simulink model "S_EXP_PI_MPPT_V1"  (R2017a)
settings: Solver=FixedStepDiscrete  StartTime=0.0  StopTime=10.0  RelTol=1e-3  EnableMultiTasking=on
undefined symbols (not defined in the file or in its folder): Down, GPTRIP1SEL, GPTRIP2SEL, TZ1, TZ2, Up
libraries: c2802xlib x3, c2806xlib x2, c280xlib x2, simulink x1, c2000lib x1
settings Model: ExtModeTrigDuration=8  Creator=dricl  LastModifiedBy=dricl
settings OptimizationCC: DefaultUnderspecifiedDataType=single  PassReuseOutputArgsAs=Individual arguments  MaxStackSize=512
settings DebuggingCC: ParameterTunabilityLossMsg=error
settings HardwareCC: ProdBitPerChar=16  ProdBitPerInt=16  ProdBitPerPointer=32  ProdBitPerSizeT=32  ProdBitPerPtrDiffT=32  ProdLargestAtomicInteger=Integer  ProdLargestAtomicFloat=None  ProdWordSize=16  ProdLongLongMode=on  ProdHWDeviceType=Texas Instruments->C2000
settings SFSimCC: MATLABDynamicMemAlloc=off
settings RTWCC: SystemTargetFile=ert.tlc  HardwareBoard=TI Piccolo F2806x  TLCOptions=-aInlineSetEventsForThisBaseRateFcn=TLC_FALSE -aSuppressMultiTaskScheduler=TLC_FALSE -aRateBasedStepFcn=1  TemplateMakefile=ert_default_tmf  Description=Embedded Coder  Toolchain=Texas Instruments Code Composer Studio v5 (C2000)  CodeExecutionProfiling=on  CodeProfilingSaveOptions=AllData  CodeProfilingInstrumentation=on
settings CodeAppCC: ForceParamTrailComments=on  IgnoreCustomStorageClasses=off  OperatorAnnotations=on  SimulinkDataObjDesc=on  SFDataObjDesc=on  MATLABFcnDesc=on  InsertBlockDesc=on  MATLABSourceComments=on
settings ERTTargetCC: CodeReplacementLibrary=TI C28x  MemSecPackage=tic2000demospkg  MemSecFuncExecute=code_ramfuncs

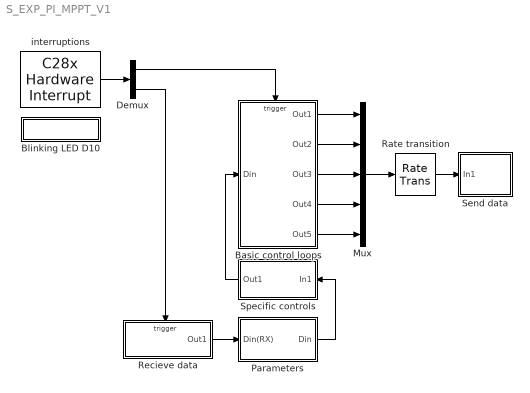
== system S_EXP_PI_MPPT_V1 ==
  Basic control loops : Subsystem  TreatAsAtomicUnit=on
      settings: RTWSystemCode=Nonreusable function
  Blinking LED D10 : Subsystem
  Demux : Demux  Outputs=2
  Mux : Mux  Inputs=5
  Parameters : Subsystem  TreatAsAtomicUnit=on
  Rate transition : RateTransition  Integrity=off  Deterministic=off  OutPortSampleTime=1/5e3
  Recieve data : Subsystem  SystemSampleTime=1e-3
      settings: RTWSystemCode=Nonreusable function
  Send data : Subsystem  TreatAsAtomicUnit=on
  Specific controls : Subsystem  TreatAsAtomicUnit=on
  interruptions : c2000lib/Scheduling/C28x Hardware Interrupt  irqnumbers=[1 9]  pienumbers=[1 1]  irqpriorities=[30 50]  irqpreempts=[1 0]  showinput=off  dspchiptype=C280X
      settings: SourceProductName=Embedded Coder Support Package for Texas Instruments C2000 Processors  SourceProductBaseCode=TIC2000
  wires:
  interruptions/1 -> Demux/1
  Demux/2 -> Recieve data/Trigger
  Recieve data/1(Out1) -> Parameters/1(Din(RX))
  Demux/1 -> Basic control loops/Trigger
  Parameters/1(Din) -> Specific controls/1(In1)
  Specific controls/1(Out1) -> Basic control loops/1(Din)
  Rate transition/1 -> Send data/1(In1)
  Mux/1 -> Rate transition/1
  Basic control loops/1(Out1) -> Mux/1
  Basic control loops/2(Out2) -> Mux/2
  Basic control loops/3(Out3) -> Mux/3
  Basic control loops/4(Out4) -> Mux/4
  Basic control loops/5(Out5) -> Mux/5

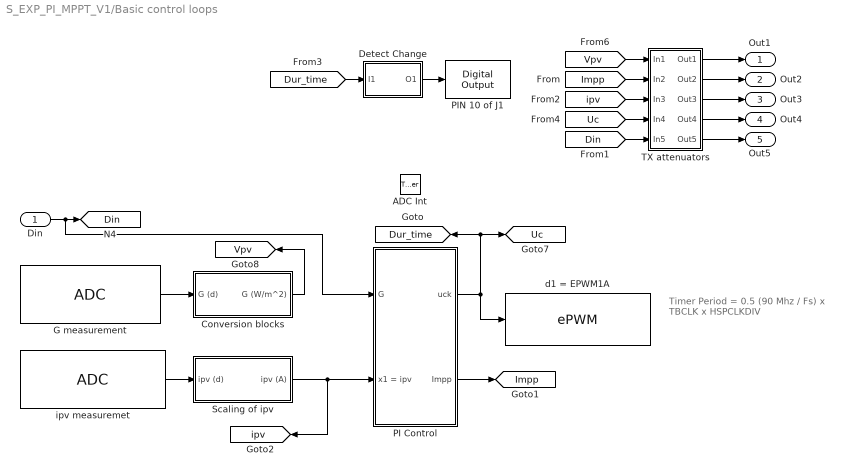
== system S_EXP_PI_MPPT_V1/Basic control loops ==
  note: Timer Period =
      |  0.5 (90 Mhz / Fs)  x
      | TBCLK x HSPCLKDIV
  Din : Inport
  ADC Int : TriggerPort  TriggerType=function-call  VariantControl=Variant
  Conversion blocks : Subsystem  Priority=5  TreatAsAtomicUnit=on
  Detect Change : Subsystem  TreatAsAtomicUnit=on
  G measurement : c2802xlib/ADC  ADCModule=1  samplingMode=Single sample mode  ADCResolution=12-bit (Single-ended input)  useSOC1=SOC1  useSOC2=SOC0_SOC1  SOCAcquisitionWindow=7  SOCTriggerSource=ePWM1_ADCSOCA  SOCInterruptTrigger=No ADCINT  Ts=-1  dType=uint16  postInterrupt=off  interruptSel=ADCINT1  ADCINTContinuous=on  endma=off  chdma=1  blkParamProc=C2000  conv1=ADCINA1  conv2=ADCINA0 and ADCINB0  conv1_Type4=ADCIN0  conv2_Type4=ADCIN0 and ADCIN1
      settings: SourceProductName=Embedded Coder Support Package for Texas Instruments C2000 Processors
  PI Control : Subsystem  Priority=7
  PIN 10 of J1 : c2806xlib/Digital Output  GPIO_Number=GPIO32~GPIO39  GPIO_Bit0=on  GPIO_BIT0_Toggle=off  GPIO_Bit1=off  GPIO_BIT1_Toggle=off  GPIO_Bit2=off  GPIO_BIT2_Toggle=off  GPIO_Bit3=off  GPIO_BIT3_Toggle=off  GPIO_Bit4=off  GPIO_BIT4_Toggle=off  GPIO_Bit5=off  GPIO_BIT5_Toggle=off  GPIO_Bit6=off  GPIO_BIT6_Toggle=off  GPIO_Bit7=off  GPIO_BIT7_Toggle=off
      settings: SourceProductName=Embedded Coder Support Package for Texas Instruments C2000 Processors  SourceProductBaseCode=TIC2000
  Scaling of ipv : Subsystem  Priority=6  TreatAsAtomicUnit=on
  TX attenuators : Subsystem  TreatAsAtomicUnit=on
  d1 = EPWM1A : c2802xlib/ePWM  useModule=ePWM1  ePWMxLINKTBPRD=Not Linked  periodUnits=Clock cycles  timerSource=Specify via dialog  timerPeriod_clk=9000  timerPeriod_sec=0.0001  tbshadow=Counter equals to zero  countingMode=Up-Down  phaseActiveEnable=Disable  phaseDirection=Count down after sync  phaseActive=0  synchronizationEnable=off  dcaevt1Sync=off  dcbevt1Sync=off  synchronizationOption=Disable  clockPrescale=1  HSclockPrescale=1  enswap=off  ePWMxAStatus=on  ePWMxAactionLogic1=Do nothing  ePWMxAactionLogic2=Do nothing  ePWMxAactionLogic3=Clear  ePWMxAactionLogic4=Set  ePWMxAactionLogic5=Do nothing  ePWMxAactionLogic6=Do nothing  ePWMxALoadMode=Load on counter equals to zero (CTR=Zero)  ePWMxACSFenable=off  ePWMxACSFvalue=Forcing disable  ePWMxASFreload=Zero  ePWMxBStatus=off  ePWMxBactionLogic1=Set  ePWMxBactionLogic2=Clear  ePWMxBactionLogic3=Do nothing  ePWMxBactionLogic4=Do nothing  ePWMxBactionLogic5=Clear  ePWMxBactionLogic6=Set  ePWMxBLoadMode=Load on counter equals to zero (CTR=Zero)  ePWMxBCSFenable=off  ePWMxBCSFvalue=Forcing disable  ePWMxBSFreload=Zero  ePWNxBOutWay=off  ePWMxLINKCMPA=Not Linked  CMPAUnits=Clock cycles  CMPASource=Input port  CMPAValue_per=50  CMPAValue_clk=9000/2  enCMPAshadow=Counter equals to zero  ePWMxLINKCMPB=Not Linked  CMPBUnits=Clock cycles  CMPBSource=Specify via dialog  CMPBValue_per=50  CMPBValue_clk=9000/2  enCMPBshadow=Counter equals to zero  ePWMxLINKCMPC=Not Linked  CMPCUnits=Clock cycles  CMPCSource=Specify via dialog  CMPCValue_per=50  CMPCValue_clk=32000  enCMPCshadow=Counter equals to zero  ePWMxLINKCMPD=Not Linked  CMPDUnits=Clock cycles  CMPDSource=Specify via dialog  CMPDValue_per=50  CMPDValue_clk=32000  enCMPDshadow=Counter equals to zero  enableDBePWMxA=on  enableDBePWMxB=on  enhalfcycle=off  DBpolarity=Active high complementary (AHC)  DBedgeDelay=Positive  DBSource_ePWMxA=ePWMxA  DBSource_ePWMxB=ePWMxA  DBperiodSource=Specify via dialog  REDperiod=50  FEDperiod=50  adcstartModuleA=on  adcrequestEventA=First event  adcstartEventA=Counter equals to period (CTR=PRD)  adcstartEventA_type2=Digital Compare Module A Event 1 start of conversion (DCAEVT1.soc)  adcstartModuleB=off  adcrequestEventB=First event  adcstartEventB=Counter equals to zero (CTR=Zero)  adcstartEventB_type2=Counter equals to zero (CTR=Zero)  intEn=off  intPrd=First event  intSel=Counter equals to zero (CTR=Zero)  intSel_type2=Counter equals to zero (CTR=Zero)  hrpe=off  enHRPWM=off  HRPWM_LoadMode=Counter equals to period (CTR=PRD)  HRPWM_CTLMode=Duty or Period control mode  HRPWM_EDGMode=Both edge  hrpeb=off  enHRPWMB=off  HRPWM_LoadModeB=Counter equals to zero (CTR=ZERO)  HRPWM_CTLModeB=Duty or Period control mode  HRPWM_EDGModeB=Both edge  enSFO=on  enautoconv=on  chopperEnable=off  chopperFrequency=1  chopperFirstwidth=1  chopperDuty=12.5%  tripZonesource=Specify via dialog  tzselOSHT1=off  tzselOSHT2=off  tzselOSHT3=off  tzselOSHDCAEV1=off  tzselOSHDCBEV1=off  tzselCBC1=off  tzselCBC2=off  tzselCBC3=off  tzselCBCDCAEV2=off  tzselCBCDCBEV2=off  tzselOSHT4=off  tzselOSHT5=off  tzselOSHT6=off  tzselCBC4=off  tzselCBC5=off  tzselCBC6=off  enTzOstIntr=off  enTzCbcIntr=off  enTzDCAEVT1Intr=off  enTzDCAEVT2Intr=off  enTzDCBEVT1Intr=off  enTzDCBEVT2Intr=off  ePWMxAforced=No action  ePWMxBforced=No action  DCAEVT1forced=No action  DCBEVT1forced=No action  DCAEVT2forced=No action  DCBEVT2forced=No action  dcah=Trip Zone 1 input (TZ1)  dcal=Trip Zone 2 input (TZ2)  dcbh=Trip Zone 1 input (TZ1)  dcbl=Trip Zone 2 input (TZ2)  dcah_type2=GPTRIP1SEL/(TZ1)  dcal_type2=GPTRIP2SEL/(TZ2)  dcbh_type2=GPTRIP1SEL/(TZ1)  dcbl_type2=GPTRIP2SEL/(TZ2)  gendcaevt1=Event disabled  gendcaevt2=Event disabled  gendcbevt1=Event disabled  gendcbevt2=Event disabled  dcaevt1src=DCAEVT1 with sync  dcaevt2src=DCAEVT2 with sync  dcbevt1src=DCBEVT1 with sync  dcbevt2src=DCBEVT2 with sync  pulsesel=Counter equals to zero (CTR=Zero)  blankinv=off  blankoffset=0  blankwidth=0  evsrcsel=Filtered version of DCAEVT1 (DCAEVT1FILT)  encape=off  PwmType=C2000
      settings: SourceProductName=Embedded Coder Support Package for Texas Instruments C2000 Processors
  ipv measuremet : c2802xlib/ADC  ADCModule=1  samplingMode=Single sample mode  ADCResolution=12-bit (Single-ended input)  useSOC1=SOC2  useSOC2=SOC0_SOC1  SOCAcquisitionWindow=7  SOCTriggerSource=ePWM1_ADCSOCA  SOCInterruptTrigger=No ADCINT  Ts=-1  dType=uint16  postInterrupt=on  interruptSel=ADCINT1  ADCINTContinuous=on  endma=off  chdma=1  blkParamProc=C2000  conv1=ADCINA0  conv2=ADCINA0 and ADCINB0  conv1_Type4=ADCIN0  conv2_Type4=ADCIN0 and ADCIN1
      settings: SourceProductName=Embedded Coder Support Package for Texas Instruments C2000 Processors
  Out1 : Outport
  Out2 : Outport  Port=2
  Out3 : Outport  Port=3
  Out4 : Outport  Port=4
  Out5 : Outport  Port=5
  tag scope: Din=global, Dur_time=global, Impp=global, Uc=global, Vpv=global, ipv=global
  wires:
  Din/1 -> PI Control/1(G), [Din]
  ipv measuremet/1 -> Scaling of ipv/1(ipv (d))
  Scaling of ipv/1(ipv (A)) -> [ipv], PI Control/2(x1 = ipv)
  TX attenuators/1(Out1) -> Out1/1
  TX attenuators/3(Out3) -> Out3/1
  TX attenuators/2(Out2) -> Out2/1
  TX attenuators/4(Out4) -> Out4/1
  [Dur_time] -> Detect Change/1(I1)
  Detect Change/1(O1) -> PIN 10 of J1/1
  G measurement/1 -> Conversion blocks/1(G (d))
  PI Control/2(Impp) -> [Impp]
  [ipv] -> TX attenuators/3(In3)
  [Impp] -> TX attenuators/2(In2)
  [Vpv] -> TX attenuators/1(In1)
  [Uc] -> TX attenuators/4(In4)
  [Din] -> TX attenuators/5(In5)
  TX attenuators/5(Out5) -> Out5/1
  PI Control/1(uck) -> d1 = EPWM1A/1, [Dur_time], [Uc]
  Conversion blocks/1(G (W/m^2)) -> [Vpv]

== system S_EXP_PI_MPPT_V1/Blinking LED D10 ==
  LED D10 : c2806xlib/Digital Output  GPIO_Number=GPIO32~GPIO39  GPIO_Bit0=off  GPIO_BIT0_Toggle=off  GPIO_Bit1=off  GPIO_BIT1_Toggle=off  GPIO_Bit2=off  GPIO_BIT2_Toggle=on  GPIO_Bit3=off  GPIO_BIT3_Toggle=off  GPIO_Bit4=off  GPIO_BIT4_Toggle=off  GPIO_Bit5=off  GPIO_BIT5_Toggle=off  GPIO_Bit6=off  GPIO_BIT6_Toggle=off  GPIO_Bit7=on  GPIO_BIT7_Toggle=on
      settings: SourceProductName=Embedded Coder Support Package for Texas Instruments C2000 Processors  SourceProductBaseCode=TIC2000
  Pulse Generator : DiscretePulseGenerator  PulseType=Time based  Period=0.25  PulseWidth=50
  wires:
  Pulse Generator/1 -> LED D10/1

== system S_EXP_PI_MPPT_V1/Parameters ==
  Din(RX) : Inport
  Attenuator 1 : Gain  Gain=20/4095  OutDataTypeStr=double
  Data Type Conversion3 : DataTypeConversion  OutDataTypeStr=double
  Rate Transition 3 : RateTransition  Integrity=off  Deterministic=off  OutPortSampleTime=0.01
  Din : Outport
  wires:
  Attenuator 1/1 -> Din/1
  Rate Transition 3/1 -> Data Type Conversion3/1
  Data Type Conversion3/1 -> Attenuator 1/1
  Din(RX)/1 -> Rate Transition 3/1

== system S_EXP_PI_MPPT_V1/Recieve data ==
  SCI_Rx_INT : TriggerPort  TriggerType=function-call  VariantControl=Variant
  SCI Receive : c280xlib/SCI Receive  sciModule=A  dataHead=''  dataTail=''  dataType=uint16  dataDim=1  initValue=0  errOption=Output the last received value  errValue=0  sampleTime=-1  outputStatus=off  postInterrupt=on  numFifo=4
      settings: SourceProductName=Embedded Coder Support Package for Texas Instruments C2000 Processors  SourceProductBaseCode=TIC2000
  Out1 : Outport  InitialOutput=[((100)*(4095/100))]
  wires:
  SCI Receive/1 -> Out1/1

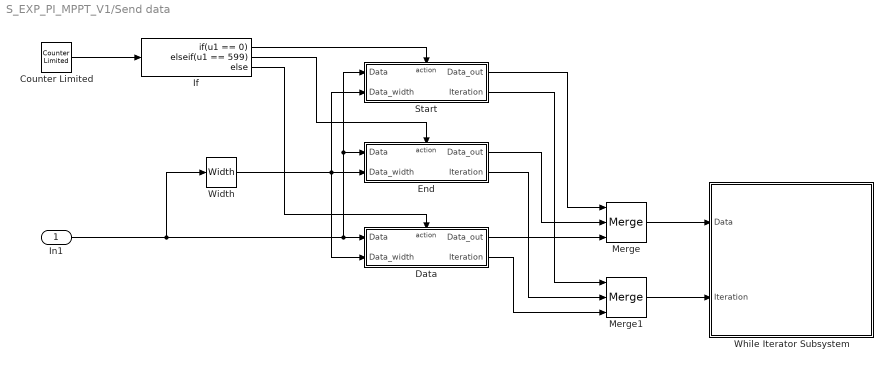
== system S_EXP_PI_MPPT_V1/Send data ==
  In1 : Inport
  Counter Limited : simulink/Sources/Counter Limited  uplimit=599  tsamp=-1
  Data : Subsystem  TreatAsAtomicUnit=on
  End : Subsystem  TreatAsAtomicUnit=on
  If : If  IfExpression=u1 == 0  ElseIfExpressions=u1 == 599
  Merge : Merge  Inputs=3
  Merge1 : Merge  Inputs=3
  Start : Subsystem  TreatAsAtomicUnit=on
  While Iterator Subsystem : Subsystem  TreatAsAtomicUnit=on
  Width : Width  OutDataTypeMode=All ports same datatype  DataType=uint16
  wires:
  If/1 -> Start/Action
  If/2 -> End/Action
  If/3 -> Data/Action
  Counter Limited/1 -> If/1
  Start/1(Data_out) -> Merge/1
  End/1(Data_out) -> Merge/2
  Data/1(Data_out) -> Merge/3
  Merge/1 -> While Iterator Subsystem/1(Data)
  Merge1/1 -> While Iterator Subsystem/2(Iteration)
  Start/2(Iteration) -> Merge1/1
  End/2(Iteration) -> Merge1/2
  Data/2(Iteration) -> Merge1/3
  In1/1 -> Width/1, Start/1(Data), End/1(Data), Data/1(Data)
  Width/1 -> Data/2(Data_width), Start/2(Data_width), End/2(Data_width)

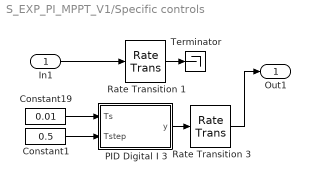
== system S_EXP_PI_MPPT_V1/Specific controls ==
  In1 : Inport
  Constant1 : Constant  Value=0.5  SampleTime=-1
  Constant19 : Constant  Value=0.01  SampleTime=-1
  PID Digital I 3 : MATLAB Function  TreatAsAtomicUnit=on
  Rate Transition 1 : RateTransition  Deterministic=off
  Rate Transition 3 : RateTransition  Deterministic=off
  Terminator : Terminator
  Out1 : Outport
  wires:
  In1/1 -> Rate Transition 1/1
  Rate Transition 1/1 -> Terminator/1
  PID Digital I 3/1(y) -> Rate Transition 3/1
  Rate Transition 3/1 -> Out1/1
  Constant19/1 -> PID Digital I 3/1(Ts)
  Constant1/1 -> PID Digital I 3/2(Tstep)

== system S_EXP_PI_MPPT_V1/Basic control loops/Conversion blocks ==
  G (d) : Inport
  Data Type Conversion2 : DataTypeConversion  OutDataTypeStr=double
  Irr (w/m^2) = Irr (d) x (30 w/m^2 / 4095 d) : Gain  Gain=30/4095
  G (W/m^2) : Outport
  wires:
  G (d)/1 -> Data Type Conversion2/1
  Data Type Conversion2/1 -> Irr (w/m^2) = Irr (d) x (30 w/m^2 / 4095 d)/1
  Irr (w/m^2) = Irr (d) x (30 w/m^2 / 4095 d)/1 -> G (W/m^2)/1

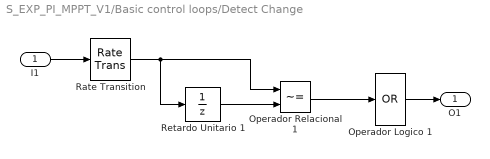
== system S_EXP_PI_MPPT_V1/Basic control loops/Detect Change ==
  I1 : Inport
  Operador Logico 1 : Logic  Operator=OR  Inputs=1  AllPortsSameDT=off  OutDataTypeStr=boolean
  Operador Relacional 1 : RelationalOperator  Operator=~=  OutDataTypeStr=boolean  RndMeth=Nearest
  Rate Transition : RateTransition  Deterministic=off
  Retardo Unitario 1 : UnitDelay  InitialCondition=0.5  SampleTime=-1
  O1 : Outport
  wires:
  Retardo Unitario 1/1 -> Operador Relacional 1/2
  I1/1 -> Rate Transition/1
  Operador Relacional 1/1 -> Operador Logico 1/1
  Operador Logico 1/1 -> O1/1
  Rate Transition/1 -> Operador Relacional 1/1, Retardo Unitario 1/1

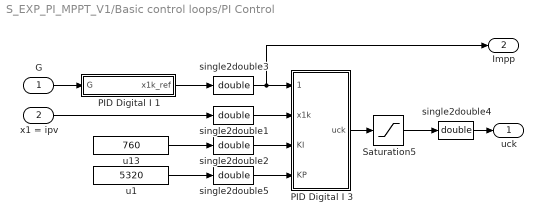
== system S_EXP_PI_MPPT_V1/Basic control loops/PI Control ==
  G : Inport
  x1 = ipv : Inport  Port=2
  PID Digital I 1 : MATLAB Function  TreatAsAtomicUnit=on
  PID Digital I 3 : MATLAB Function  TreatAsAtomicUnit=on
  Saturation5 : Saturate  UpperLimit=9000*0.98  LowerLimit=9000*0.05
  single2double{1..5} (5 alike) : DataTypeConversion  OutDataTypeStr=double
  u1 : Constant  Value=5320  SampleTime=-1
  u13 : Constant  Value=760  SampleTime=-1
  uck : Outport
  Impp : Outport  Port=2
  wires:
  u1/1 -> single2double5/1
  u13/1 -> single2double2/1
  G/1 -> PID Digital I 1/1(G)
  single2double3/1 -> Impp/1, PID Digital I 3/1(x1k_ref)
  single2double1/1 -> PID Digital I 3/2(x1k)
  Saturation5/1 -> single2double4/1
  single2double4/1 -> uck/1
  single2double2/1 -> PID Digital I 3/3(KI)
  single2double5/1 -> PID Digital I 3/4(KP)
  x1 = ipv/1 -> single2double1/1
  PID Digital I 3/1(uck) -> Saturation5/1
  PID Digital I 1/1(x1k_ref) -> single2double3/1

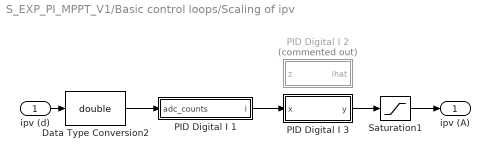
== system S_EXP_PI_MPPT_V1/Basic control loops/Scaling of ipv ==
  ipv (d) : Inport
  Data Type Conversion2 : DataTypeConversion  OutDataTypeStr=double
  PID Digital I 1 : MATLAB Function  TreatAsAtomicUnit=on
  PID Digital I 2 : MATLAB Function  Commented=on  TreatAsAtomicUnit=on
  PID Digital I 3 : MATLAB Function  TreatAsAtomicUnit=on
  Saturation1 : Saturate  UpperLimit=inf  LowerLimit=0
  ipv (A) : Outport
  wires:
  ipv (d)/1 -> Data Type Conversion2/1
  Data Type Conversion2/1 -> PID Digital I 1/1(adc_counts)
  Saturation1/1 -> ipv (A)/1
  PID Digital I 1/1(i) -> PID Digital I 3/1(x)
  PID Digital I 3/1(y) -> Saturation1/1

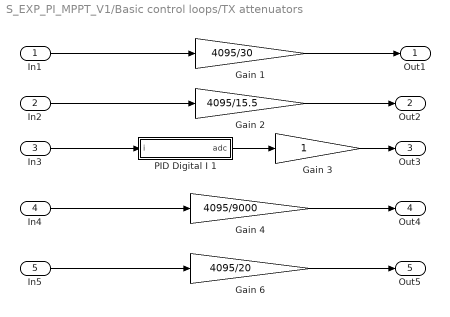
== system S_EXP_PI_MPPT_V1/Basic control loops/TX attenuators ==
  In1 : Inport
  In2 : Inport  Port=2
  In3 : Inport  Port=3
  In4 : Inport  Port=4
  In5 : Inport  Port=5
  Gain 1 : Gain  Gain=4095/30  OutDataTypeStr=uint16  RndMeth=Simplest
  Gain 2 : Gain  Gain=4095/15.5  OutDataTypeStr=uint16  RndMeth=Simplest
  Gain 3 : Gain  OutDataTypeStr=uint16  RndMeth=Simplest
  Gain 4 : Gain  Gain=4095/9000  OutDataTypeStr=uint16  RndMeth=Simplest
  Gain 6 : Gain  Gain=4095/20  OutDataTypeStr=uint16  RndMeth=Simplest
  PID Digital I 1 : MATLAB Function  TreatAsAtomicUnit=on
  Out1 : Outport
  Out2 : Outport  Port=2
  Out3 : Outport  Port=3
  Out4 : Outport  Port=4
  Out5 : Outport  Port=5
  wires:
  PID Digital I 1/1(adc) -> Gain 3/1
  In4/1 -> Gain 4/1
  Gain 4/1 -> Out4/1
  Gain 2/1 -> Out2/1
  In2/1 -> Gain 2/1
  In3/1 -> PID Digital I 1/1(i)
  Gain 3/1 -> Out3/1
  In1/1 -> Gain 1/1
  Gain 1/1 -> Out1/1
  In5/1 -> Gain 6/1
  Gain 6/1 -> Out5/1

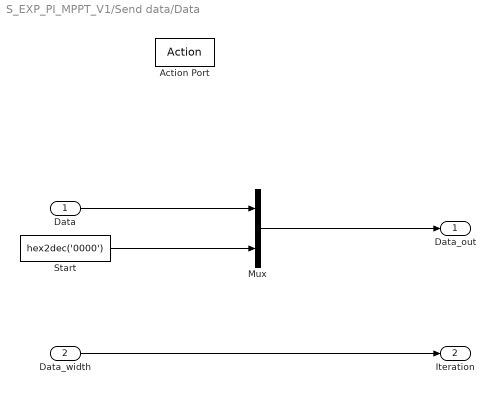
== system S_EXP_PI_MPPT_V1/Send data/Data ==
  Data : Inport
  Data_width : Inport  Port=2
  Action Port : ActionPort  ActionType=else
  Mux : Mux  Inputs=2
  Start : Constant  Value=hex2dec('0000')  OutDataTypeStr=uint16
  Data_out : Outport
  Iteration : Outport  Port=2
  wires:
  Start/1 -> Mux/2
  Mux/1 -> Data_out/1
  Data/1 -> Mux/1
  Data_width/1 -> Iteration/1

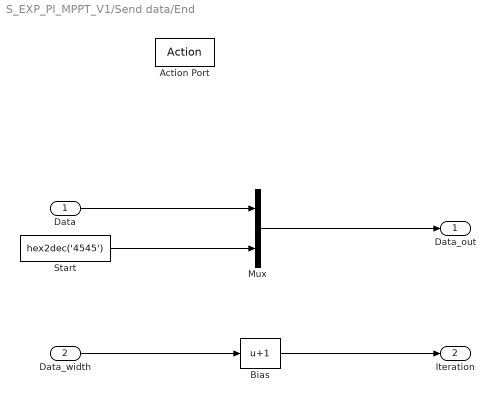
== system S_EXP_PI_MPPT_V1/Send data/End ==
  Data : Inport
  Data_width : Inport  Port=2
  Action Port : ActionPort  ActionType=elseif
  Bias : Bias  Bias=1
  Mux : Mux  Inputs=2
  Start : Constant  Value=hex2dec('4545')  OutDataTypeStr=uint16
  Data_out : Outport
  Iteration : Outport  Port=2
  wires:
  Mux/1 -> Data_out/1
  Data_width/1 -> Bias/1
  Start/1 -> Mux/2
  Bias/1 -> Iteration/1
  Data/1 -> Mux/1

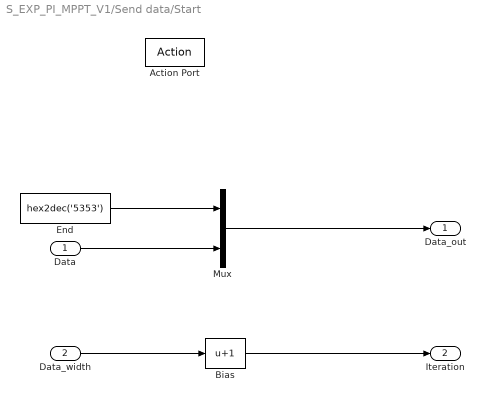
== system S_EXP_PI_MPPT_V1/Send data/Start ==
  Data : Inport
  Data_width : Inport  Port=2
  Action Port : ActionPort  ActionType=then
  Bias : Bias  Bias=1
  End : Constant  Value=hex2dec('5353')  OutDataTypeStr=uint16
  Mux : Mux  Inputs=2
  Data_out : Outport
  Iteration : Outport  Port=2
  wires:
  End/1 -> Mux/1
  Mux/1 -> Data_out/1
  Data_width/1 -> Bias/1
  Bias/1 -> Iteration/1
  Data/1 -> Mux/2

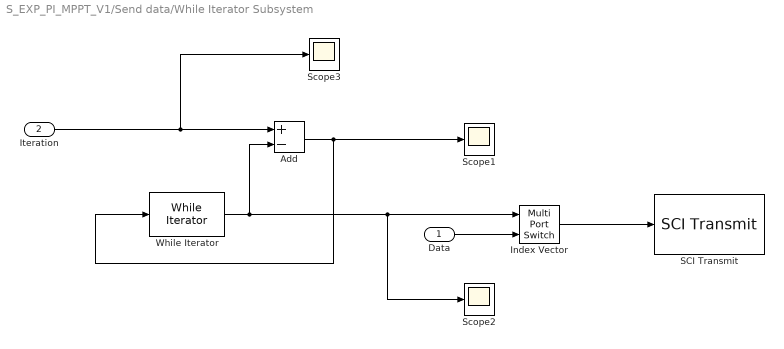
== system S_EXP_PI_MPPT_V1/Send data/While Iterator Subsystem ==
  Data : Inport
  Iteration : Inport  Port=2
  Add : Sum  Inputs=+-  OutDataTypeStr=Inherit: Same as first input
  Index Vector : MultiPortSwitch  Inputs=1
  SCI Transmit : c280xlib/SCI Transmit  sciModule=A  dataHead=''  dataTail=''  postInterrupt=off  numFifo=1
      settings: SourceProductName=Embedded Coder Support Package for Texas Instruments C2000 Processors
  Scope1 : Scope
  Scope2 : Scope
  Scope3 : Scope
  While Iterator : WhileIterator  MaxIters=-1  WhileBlockType=do-while  ShowIterationPort=on  OutputDataType=int16
  wires:
  Iteration/1 -> Scope3/1, Add/1
  Add/1 -> Scope1/1, While Iterator/1
  Index Vector/1 -> SCI Transmit/1
  Data/1 -> Index Vector/2
  While Iterator/1 -> Scope2/1, Index Vector/1, Add/2

== matlab function S_EXP_PI_MPPT_V1/Basic control loops/Scaling of ipv/PID Digital I 2 ==
  data: z input; ihat output
function ihat = fcn(z)
% Kalman 2D para ipv: estima i y di/dt
Ts = 1/5000;

A = [1 Ts; 0 1];
C = [1 0];

% Ajuste inicial (suaviza bien sin matar dinámica)
q_i  = 1e-7;
q_di = 1e-2;
Q = [q_i 0; 0 q_di];

R = 5e-3;  % sube a 1e-2 si aún tiembla

persistent x P
if isempty(x)
    x = [z; 0];
    P = eye(2);
end

% Predict
x_pred = A*x;
P_pred = A*P*A' + Q;

% Update
S = C*P_pred*C' + R;
K = (P_pred*C')/S;

x = x_pred + K*(z - C*x_pred);
P = (eye(2) - K*C)*P_pred;

ihat = x(1);
end

== matlab function S_EXP_PI_MPPT_V1/Basic control loops/TX attenuators/PID Digital I 1 ==
  data: i input; adc output
function adc = fcn(i)
% Corriente corregida (A) -> ADC (0..4095)

ADCmax = 4095;

% Misma calibración
m = 2/1.85;                 
c = 0.5405405405405406;

% Inversa: i_raw = (i - c)/m
i_raw = (double(i) - c) / m;

% i_raw = 36.7*(adc/4095) - 18.3  ->  adc = 4095*((i_raw+18.3)/36.7)
adc = ADCmax * ((i_raw + 18.3) / 36.7);

% Saturación
if adc > ADCmax
    adc = ADCmax;
elseif adc < 0
    adc = 0;
end

adc = round(adc);

end

== matlab function S_EXP_PI_MPPT_V1/Basic control loops/Scaling of ipv/PID Digital I 1 ==
  data: adc_counts input; i output
function i = fcn(adc_counts)
% adc_counts: 0..4095
% i: corriente corregida (A)

ADCmax = 4095;

% Conversión ideal (datasheet)
i_raw = 36.7 * (double(adc_counts)/double(ADCmax)) - 18.3;

% Calibración con tus 2 puntos:
% i_raw(0A)=-0.5  y  i_raw(2A)=1.35
m = 2/1.85;                 % 1.081081081...
c = 0.5405405405405406;     % = m*0.5

i = m*i_raw + c;

% Saturación opcional
if i > 15.5
    i = 15.5;
elseif i < -15.5
    i = -15.5;
end

end

== matlab function S_EXP_PI_MPPT_V1/Basic control loops/PI Control/PID Digital I 1 ==
  data: G input; x1k_ref output
function x1k_ref = fcn(G)

% Generador de referencia i_mpp (Opción B ajustada)
% G : equivalente a Vs (V)
% x1k_ref : referencia de corriente (A)

% Parametros del mapeo para G en [6,10] V -> i_mpp en [0.5,2] A
m = 0.375;
b = -1.75;

% Calculo de la referencia
x1k_ref = m*G + b;

% Saturacion de seguridad
if x1k_ref > 2.5
    x1k_ref = 2.5;
end

if x1k_ref < 0.0
    x1k_ref = 0.0;
end

end

== matlab function S_EXP_PI_MPPT_V1/Basic control loops/Scaling of ipv/PID Digital I 3 ==
  data: x input; y output
function y = fcn(x)
% Filtro 1er orden pasa-bajas: H(s)=a/(s+a)
% Discretización: Euler hacia atrás (implícito)
% x: señal medida (ej. ipv)
% y: señal filtrada

Ts = 1/5000;     % periodo de muestreo
fc = 20;         % Hz (ajusta)
a  = 2*pi*fc;    % rad/s

persistent yk
if isempty(yk)
    yk = x;      % inicializa con la medición para evitar salto
end

% Euler hacia atrás:
% y[k] = ( y[k-1] + Ts*a*x[k] ) / (1 + Ts*a)
yk = (yk + Ts*a*x) / (1 + Ts*a);

y = yk;
end

== matlab function S_EXP_PI_MPPT_V1/Basic control loops/PI Control/PID Digital I 3 ==
  data: x1k_ref input; uck output; x1k input; KI input; KP input
function uck = fcn(x1k_ref, x1k, KI, KP)

 %Valores iniciales de las conStantes del controlador
 persistent  ek uk
 persistent  ek_1 uk_1
 if isempty(ek)
    ek =0;
    uk =0;
    ek_1 =0;
    uk_1 =0;
 end
ek=x1k_ref-x1k;
uk=ek*(KP+KI)-ek_1*KP+uk_1;
%uk=KP*ek+KI*ek+KI*ek_1;
% if(uk>(1*65535))
%     uk=1*65535;
% end
% if(uk<0)
%     uk=0;
% end
ek_1=ek;
uk_1=uk;
uck=uk;
end

== matlab function S_EXP_PI_MPPT_V1/Specific controls/PID Digital I 3 ==
  data: y output; Ts input; Tstep input
function y = fcn(Ts, Tstep)
% Generador discreto de niveles con duración ajustable
% Ts    : tiempo de muestreo real del bloque
% Tstep : duración de cada nivel (segundos)

levels = [0 11 6 10 8];

Nstep   = max(1, round(Tstep/Ts));
Nlevels = numel(levels);

persistent n
if isempty(n)
    n = 0;
end

idx = floor(n / Nstep);
idx = mod(idx, Nlevels) + 1;

y = levels(idx);

n = n + 1;
end
